simulink model "simulation"  (R2018a)
settings: Solver=VariableStepAuto  StartTime=0.0  StopTime=150  RelTol=1e-3
settings Model: Creator=Migue  LastModifiedBy=Migue

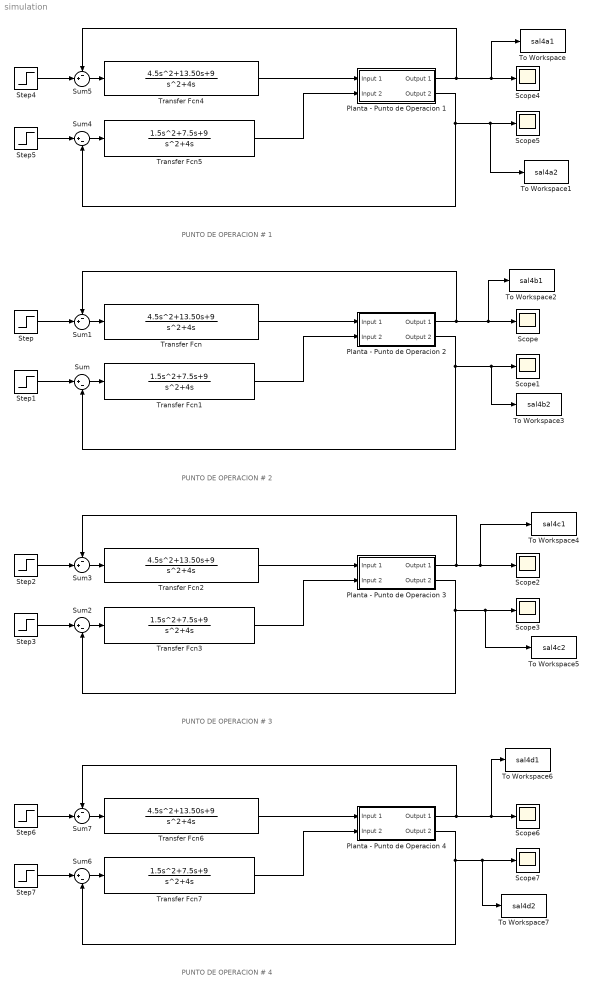
== system simulation ==
  note: PUNTO DE OPERACION # 2
  note: PUNTO DE OPERACION # 3
  note: PUNTO DE OPERACION # 1
  note: PUNTO DE OPERACION # 4
  Planta - Punto de Operacion 1 : Subsystem
  "Planta - Punto de Operacion 2 " : Subsystem
  Planta - Punto de Operacion 3 : Subsystem
  Planta - Punto de Operacion 4 : Subsystem
  Scope{,1..7} (8 alike) : Scope
  Step{,2,4,6} (4 alike) : Step  SampleTime=0
  Step{1,3,5,7} (4 alike) : Step  Time=10  After=-1  SampleTime=0
  Sum{,2,4,6} (4 alike) : Sum  Inputs=|+-
  Sum{1,3,5,7} (4 alike) : Sum  Inputs=-+|
  To Workspace : ToWorkspace  VariableName=sal4a1  SaveFormat=Timeseries  SampleTime=-1
  To Workspace1 : ToWorkspace  VariableName=sal4a2  SaveFormat=Timeseries  SampleTime=-1
  To Workspace2 : ToWorkspace  VariableName=sal4b1  SaveFormat=Timeseries  SampleTime=-1
  To Workspace3 : ToWorkspace  VariableName=sal4b2  SaveFormat=Timeseries  SampleTime=-1
  To Workspace4 : ToWorkspace  VariableName=sal4c1  SaveFormat=Timeseries  SampleTime=-1
  To Workspace5 : ToWorkspace  VariableName=sal4c2  SaveFormat=Timeseries  SampleTime=-1
  To Workspace6 : ToWorkspace  VariableName=sal4d1  SaveFormat=Timeseries  SampleTime=-1
  To Workspace7 : ToWorkspace  VariableName=sal4d2  SaveFormat=Timeseries  SampleTime=-1
  Transfer Fcn{,2,4,6} (4 alike) : TransferFcn  Numerator=[4.5 13.50 9]  Denominator=[1 4 0]
  Transfer Fcn{1,3,5,7} (4 alike) : TransferFcn  Numerator=[1.5 7.5 9]  Denominator=[1 4 0]
  wires:
  "Planta - Punto de Operacion 2 "/1(Output 1) -> Sum1/1, To Workspace2/1, Scope/1
  "Planta - Punto de Operacion 2 "/2(Output 2) -> Sum/2, To Workspace3/1, Scope1/1
  Step/1 -> Sum1/2
  Transfer Fcn/1 -> "Planta - Punto de Operacion 2 "/1(Input 1)
  Sum1/1 -> Transfer Fcn/1
  Sum/1 -> Transfer Fcn1/1
  Step1/1 -> Sum/1
  Transfer Fcn1/1 -> "Planta - Punto de Operacion 2 "/2(Input 2)
  Transfer Fcn2/1 -> Planta - Punto de Operacion 3/1(Input 1)
  Step2/1 -> Sum3/2
  Planta - Punto de Operacion 3/1(Output 1) -> Sum3/1, To Workspace4/1, Scope2/1
  Planta - Punto de Operacion 3/2(Output 2) -> Sum2/2, To Workspace5/1, Scope3/1
  Sum3/1 -> Transfer Fcn2/1
  Sum2/1 -> Transfer Fcn3/1
  Step3/1 -> Sum2/1
  Transfer Fcn3/1 -> Planta - Punto de Operacion 3/2(Input 2)
  Transfer Fcn4/1 -> Planta - Punto de Operacion 1/1(Input 1)
  Step4/1 -> Sum5/2
  Planta - Punto de Operacion 1/1(Output 1) -> Sum5/1, To Workspace/1, Scope4/1
  Planta - Punto de Operacion 1/2(Output 2) -> Sum4/2, To Workspace1/1, Scope5/1
  Sum5/1 -> Transfer Fcn4/1
  Sum4/1 -> Transfer Fcn5/1
  Step5/1 -> Sum4/1
  Transfer Fcn5/1 -> Planta - Punto de Operacion 1/2(Input 2)
  Planta - Punto de Operacion 4/1(Output 1) -> Sum7/1, To Workspace6/1, Scope6/1
  Planta - Punto de Operacion 4/2(Output 2) -> Sum6/2, To Workspace7/1, Scope7/1
  Transfer Fcn6/1 -> Planta - Punto de Operacion 4/1(Input 1)
  Sum7/1 -> Transfer Fcn6/1
  Step7/1 -> Sum6/1
  Transfer Fcn7/1 -> Planta - Punto de Operacion 4/2(Input 2)
  Sum6/1 -> Transfer Fcn7/1
  Step6/1 -> Sum7/2

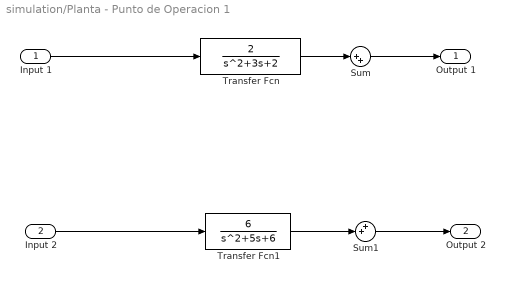
== system simulation/Planta - Punto de Operacion 1 ==
  Input 1 : Inport
  Input 2 : Inport  Port=2
  Sum : Sum  Inputs=|++
  Sum1 : Sum  Inputs=++|
  Transfer Fcn : TransferFcn  Numerator=[2]  Denominator=[1 3 2]
  Transfer Fcn1 : TransferFcn  Numerator=[6]  Denominator=[1 5 6]
  Output 1 : Outport
  Output 2 : Outport  Port=2
  wires:
  Sum1/1 -> Output 2/1
  Input 2/1 -> Transfer Fcn1/1
  Transfer Fcn/1 -> Sum/1
  Input 1/1 -> Transfer Fcn/1
  Transfer Fcn1/1 -> Sum1/2
  Sum/1 -> Output 1/1

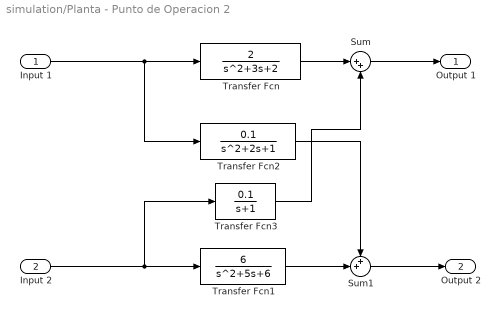
== system simulation/Planta - Punto de Operacion 2  ==
  Input 1 : Inport
  Input 2 : Inport  Port=2
  Sum : Sum  Inputs=|++
  Sum1 : Sum  Inputs=++|
  Transfer Fcn : TransferFcn  Numerator=[2]  Denominator=[1 3 2]
  Transfer Fcn1 : TransferFcn  Numerator=[6]  Denominator=[1 5 6]
  Transfer Fcn2 : TransferFcn  Numerator=[0.1]
  Transfer Fcn3 : TransferFcn  Numerator=[0.1]  Denominator=[1 1]
  Output 1 : Outport
  Output 2 : Outport  Port=2
  wires:
  Sum1/1 -> Output 2/1
  Transfer Fcn3/1 -> Sum/2
  Input 2/1 -> Transfer Fcn3/1, Transfer Fcn1/1
  Transfer Fcn/1 -> Sum/1
  Transfer Fcn2/1 -> Sum1/1
  Input 1/1 -> Transfer Fcn2/1, Transfer Fcn/1
  Transfer Fcn1/1 -> Sum1/2
  Sum/1 -> Output 1/1

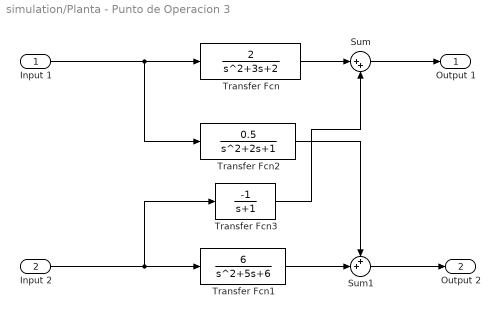
== system simulation/Planta - Punto de Operacion 3 ==
  Input 1 : Inport
  Input 2 : Inport  Port=2
  Sum : Sum  Inputs=|++
  Sum1 : Sum  Inputs=++|
  Transfer Fcn : TransferFcn  Numerator=[2]  Denominator=[1 3 2]
  Transfer Fcn1 : TransferFcn  Numerator=[6]  Denominator=[1 5 6]
  Transfer Fcn2 : TransferFcn  Numerator=[0.5]
  Transfer Fcn3 : TransferFcn  Numerator=[-1]  Denominator=[1 1]
  Output 1 : Outport
  Output 2 : Outport  Port=2
  wires:
  Sum1/1 -> Output 2/1
  Transfer Fcn3/1 -> Sum/2
  Input 2/1 -> Transfer Fcn3/1, Transfer Fcn1/1
  Transfer Fcn/1 -> Sum/1
  Transfer Fcn2/1 -> Sum1/1
  Input 1/1 -> Transfer Fcn2/1, Transfer Fcn/1
  Transfer Fcn1/1 -> Sum1/2
  Sum/1 -> Output 1/1

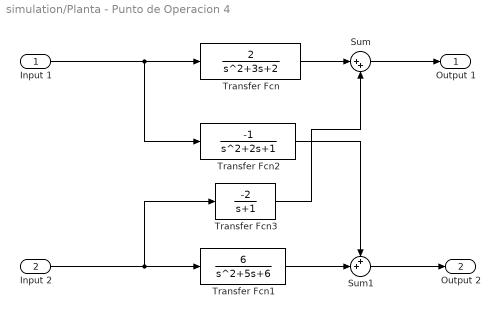
== system simulation/Planta - Punto de Operacion 4 ==
  Input 1 : Inport
  Input 2 : Inport  Port=2
  Sum : Sum  Inputs=|++
  Sum1 : Sum  Inputs=++|
  Transfer Fcn : TransferFcn  Numerator=[2]  Denominator=[1 3 2]
  Transfer Fcn1 : TransferFcn  Numerator=[6]  Denominator=[1 5 6]
  Transfer Fcn2 : TransferFcn  Numerator=[-1]
  Transfer Fcn3 : TransferFcn  Numerator=[-2]  Denominator=[1 1]
  Output 1 : Outport
  Output 2 : Outport  Port=2
  wires:
  Sum1/1 -> Output 2/1
  Transfer Fcn3/1 -> Sum/2
  Input 2/1 -> Transfer Fcn3/1, Transfer Fcn1/1
  Transfer Fcn/1 -> Sum/1
  Transfer Fcn2/1 -> Sum1/1
  Input 1/1 -> Transfer Fcn2/1, Transfer Fcn/1
  Transfer Fcn1/1 -> Sum1/2
  Sum/1 -> Output 1/1
